simulink model "vacuum_object"  (R2025a)
settings: Solver=FixedStepDiscrete  StartTime=0.0  StopTime=inf  FixedStep=0.01  RelTol=1e-3
PreLoadFcn:
  | frs = FrankaRobotSettings;
undefined symbols (not defined in the file): drop_off, dropoff_timeout, franka_default_vacuum_gripper_command, read_state, stop, vacuum, vacuum_profile, vacuum_setpoint, vacuum_timeout
libraries: franka_simulink x1
settings Model: SimulationMode=external  ExtModeTrigDuration=10000  Creator=vasi_ko  LastModifiedBy=kvasios
settings SolverCC: ConcurrentTasks=on  AlgebraicLoopSolver=TrustRegion  AutoInsertRateTranBlk=on
settings DataIOCC: LimitDataPoints=on  SaveFormat=Array  ReturnWorkspaceOutputs=off
settings OptimizationCC: EnhancedBackFolding=on  PassReuseOutputArgsAs=Individual arguments  ZeroExternalMemoryAtStartup=off  ZeroInternalMemoryAtStartup=off  MaxStackSize=200000  OptimizeBlockOrder=speed  DifferentSizesBufferReuse=on  OptimizationCustomize=off  EfficientTunableParamExpr=on
settings DebuggingCC: SolverPrmCheckMsg=warning  ParameterTunabilityLossMsg=error  UnconnectedInputMsg=warning  UnconnectedOutputMsg=warning  UnconnectedLineMsg=warning  SFUnexpectedBacktrackingDiag=warning  SFNoUnconditionalDefaultTransitionDiag=warning  SFExecutionAtInitializationDiag=none  ArithmeticOperatorsInVariantConditions=warning
settings HardwareCC: ProdBitPerLong=64.0  ProdLargestAtomicInteger=LongLong  ProdLargestAtomicFloat=Double  ProdLongLongMode=on  ProdHWDeviceType=ARM Compatible->ARM Cortex-A (64-bit)
settings ModelReferenceCC: EnableRefExpFcnMdlSchedulingChecks=on  PropagateSignalLabelsOutOfModel=off
settings SFSimCC: SimUseLocalCustomCode=off  MATLABDynamicMemAlloc=off  CustomCodeUndefinedFunction=UseInterfaceOnly  SimTargetLang=C++  SimDLTargetLibrary=mkl-dnn
settings RTWCC: SystemTargetFile=ert.tlc  HardwareBoard=NVIDIA Jetson  TLCOptions="-aInlineSetEventsForThisBaseRateFcn=TLC_FALSE -aSuppressMultiTaskScheduler=TLC_FALSE  -aRateBasedStepFcn=0"  TemplateMakefile=ert_default_tmf  RTWVerbose=off  RTWUseLocalCustomCode=off  BuildConfiguration=Faster Runs  TargetLang=C++  GPUComputeCapability=3.5  DLArmComputeVersion=19.05  Description=Embedded Coder
settings CodeAppCC: ForceParamTrailComments=on  IgnoreCustomStorageClasses=off  OperatorAnnotations=on  SimulinkDataObjDesc=on  SFDataObjDesc=on  InsertBlockDesc=on
settings ERTTargetCC: ExtModeTransport=2.0  InlinedParameterPlacement=Hierarchical  RootIOFormat=Structure reference  TargetLangStandard=C++14 (ISO)
settings ConfigComp: CovMetricSettings=dw  CovSaveCumulativeToWorkspaceVar=on  CovSaveSingleToWorkspaceVar=on  CovExternalEMLEnable=off  CovSFcnEnable=off

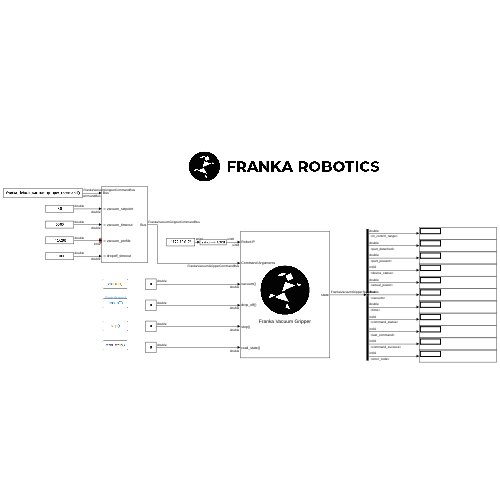
[thumbnail: Simulink's stored preview of the top-level diagram]
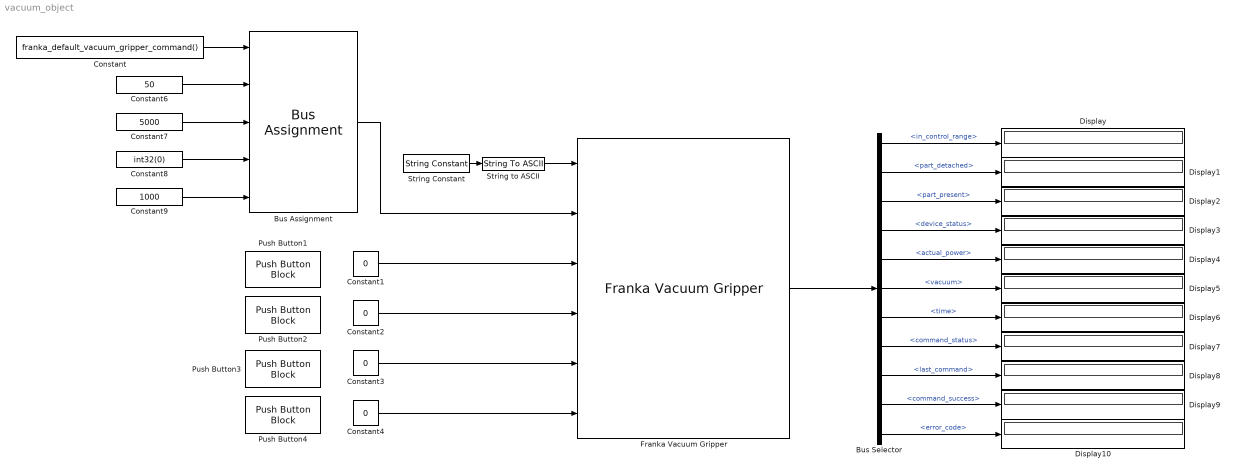
== system vacuum_object ==
  Bus Assignment : BusAssignment  AssignedSignals=vacuum_setpoint,vacuum_timeout,vacuum_profile,dropoff_timeout
  Bus Selector : BusSelector  OutputSignals=in_control_range,part_detached,part_present,device_status,actual_power,vacuum,time,command_status,last_command,command_success,error_code
  Constant : Constant  Value=franka_default_vacuum_gripper_command()  OutDataTypeStr=Bus: FrankaVacuumGripperCommandBus
  Constant{1..4} (4 alike) : Constant  Value=0
  Constant6 : Constant  Value=50
  Constant7 : Constant  Value=5000
  Constant8 : Constant  Value=int32(0)
  Constant9 : Constant  Value=1000
  Display{,1..10} (11 alike) : Display
  Franka Vacuum Gripper : franka_simulink/Franka Vacuum Gripper
      settings: SourceProductName=Franka Robotics Simulink Support Package
  Push Button1 : PushButtonBlock  ButtonText=vacuum()  IconOnColor=[0.0, 0.39215686274509803, 0.0]  IconOffColor=[0.0, 1.0, 0.0]  OffValue=0.000000
  Push Button2 : PushButtonBlock  ButtonText=drop_off()  IconOnColor=[0.0, 0.39215686274509803, 0.0]  IconOffColor=[0.0, 1.0, 0.0]  OffValue=0.000000
  Push Button3 : PushButtonBlock  ButtonText=stop()  IconOnColor=[0.0, 0.39215686274509803, 0.0]  IconOffColor=[0.0, 1.0, 0.0]  OffValue=0.000000
  Push Button4 : PushButtonBlock  ButtonText=read_state()  IconOnColor=[0.0, 0.39215686274509803, 0.0]  IconOffColor=[0.0, 1.0, 0.0]  OffValue=0.000000
  String Constant : StringConstant  String="\"172.16.0.2\""
  String to ASCII : StringToASCII  OutputVectorSize=16
  wires:
  Constant1/1 -> Franka Vacuum Gripper/3
  Constant2/1 -> Franka Vacuum Gripper/4
  Constant3/1 -> Franka Vacuum Gripper/5
  Constant4/1 -> Franka Vacuum Gripper/6
  String Constant/1 -> String to ASCII/1
  String to ASCII/1 -> Franka Vacuum Gripper/1
  Franka Vacuum Gripper/1 -> Bus Selector/1
  Bus Assignment/1 -> Franka Vacuum Gripper/2
  Constant/1 -> Bus Assignment/1
  Constant6/1 -> Bus Assignment/2
  Constant7/1 -> Bus Assignment/3
  Constant8/1 -> Bus Assignment/4
  Constant9/1 -> Bus Assignment/5
  Bus Selector/1 -> Display/1  "<in_control_range>"
  Bus Selector/2 -> Display1/1  "<part_detached>"
  Bus Selector/3 -> Display2/1  "<part_present>"
  Bus Selector/4 -> Display3/1  "<device_status>"
  Bus Selector/5 -> Display4/1  "<actual_power>"
  Bus Selector/6 -> Display5/1  "<vacuum>"
  Bus Selector/7 -> Display6/1  "<time>"
  Bus Selector/8 -> Display7/1  "<command_status>"
  Bus Selector/9 -> Display8/1  "<last_command>"
  Bus Selector/10 -> Display9/1  "<command_success>"
  Bus Selector/11 -> Display10/1  "<error_code>"
